simulink model "chap7_4sim"  (Simulink 8.1)
settings: Solver=ode45  StartTime=0.0  StopTime=10  RelTol=1e-5
settings Model: Creator=hp  LastModifiedBy=liujk  ExtModeTrigMode=oneshot  ExtModeArmWhenConnect=off
settings DataIOCC: LimitDataPoints=off  SignalLoggingName=sigsOut
settings OptimizationCC: BooleanDataType=off  InitFltsAndDblsToZero=on
settings DebuggingCC: SaveWithParameterizedLinksMsg=none  SignalResolutionControl=TryResolveAllWithWarning  SolverPrmCheckMsg=none  MultiTaskDSMMsg=warning  MultiTaskCondExecSysMsg=none  StrictBusMsg=Warning
settings HardwareCC: TargetUnknown=on
settings RTWCC: IncludeERTFirstTime=on
settings GRTTargetCC: TargetFcnLib=ansi_tfl_tmw.mat

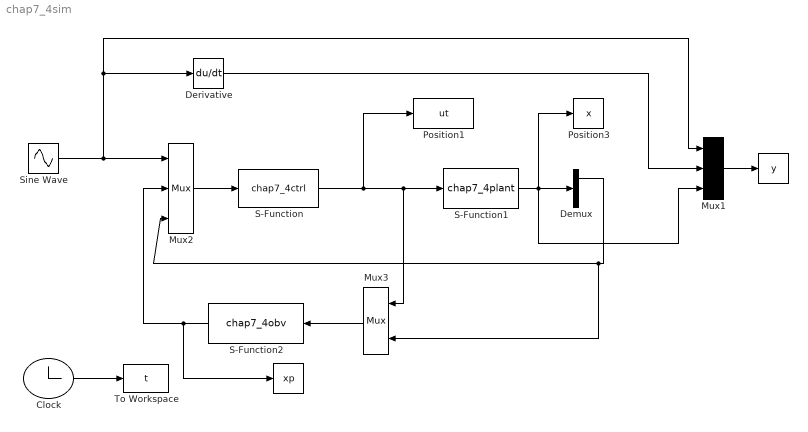
== system chap7_4sim ==
  " " : ToWorkspace  VariableName=y  SampleTime=-1
  "   " : ToWorkspace  VariableName=xp  SampleTime=-1
  Clock : Clock
  Demux : Demux  Outputs=2
  Derivative : Derivative
  Mux1 : Mux  Inputs=3
  Mux2 : Mux  Inputs=3
  Mux3 : Mux  Inputs=2
  Position1 : ToWorkspace  VariableName=ut  SampleTime=-1
  Position3 : ToWorkspace  VariableName=x  SampleTime=-1
  S-Function : S-Function  FunctionName=chap7_4ctrl  EnableBusSupport=off
  S-Function1 : S-Function  FunctionName=chap7_4plant  EnableBusSupport=off
  S-Function2 : S-Function  FunctionName=chap7_4obv  EnableBusSupport=off
  Sine Wave : Sin  SampleTime=0
  To Workspace : ToWorkspace  VariableName=t  SampleTime=-1
  wires:
  Mux1/1 -> " "/1
  Clock/1 -> To Workspace/1
  Sine Wave/1 -> Mux2/1, Mux1/1, Derivative/1
  S-Function/1 -> Position1/1, S-Function1/1, Mux3/1
  Derivative/1 -> Mux1/2
  Mux3/1 -> S-Function2/1
  Demux/1 -> Mux2/3, Mux3/2
  S-Function1/1 -> Demux/1, Position3/1, Mux1/3
  S-Function2/1 -> Mux2/2, "   "/1
  Mux2/1 -> S-Function/1
